simulink model "simple_logic_calculator"  (R2017b)
settings: Solver=FixedStepDiscrete  StartTime=0.0  StopTime=10.0  RelTol=1e-3
settings Model: Creator=ebrah  LastModifiedBy=ebrah
settings OptimizationCC: DefaultParameterBehavior=Inlined  PassReuseOutputArgsAs=Individual arguments
settings DebuggingCC: ParameterTunabilityLossMsg=error
settings SFSimCC: MATLABDynamicMemAlloc=off
settings RTWCC: SystemTargetFile=ert.tlc  GenCodeOnly=on  TemplateMakefile=ert_default_tmf  GenerateReport=on  IncludeHyperlinkInReport=on  LaunchReport=on  GenerateTraceInfo=on  GenerateTraceReport=on  GenerateTraceReportSl=on  GenerateTraceReportSf=on  GenerateTraceReportEml=on  GenerateWebview=on
settings CodeAppCC: ForceParamTrailComments=on  IgnoreCustomStorageClasses=off  OperatorAnnotations=on  SimulinkDataObjDesc=on  SFDataObjDesc=on  InsertBlockDesc=on
settings ERTTargetCC: TargetLangStandard=C99 (ISO)  GenerateSampleERTMain=on  InlinedParameterPlacement=NonHierarchical  ERTCustomFileTemplate=example_file_process.tlc

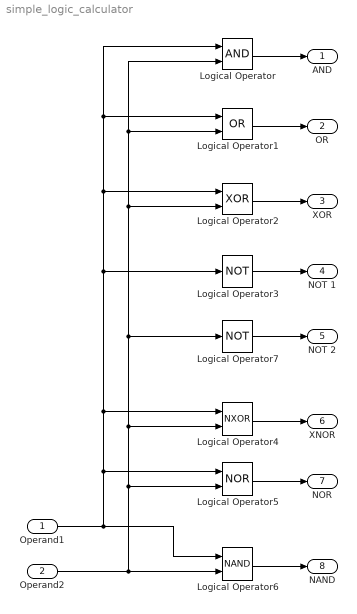
== system simple_logic_calculator ==
  Operand1 : Inport
  Operand2 : Inport  Port=2
  Logical Operator : Logic  AllPortsSameDT=off  OutDataTypeStr=boolean
  Logical Operator1 : Logic  Operator=OR  AllPortsSameDT=off  OutDataTypeStr=boolean
  Logical Operator2 : Logic  Operator=XOR  AllPortsSameDT=off  OutDataTypeStr=boolean
  Logical Operator3 : Logic  Operator=NOT  AllPortsSameDT=off  OutDataTypeStr=boolean
  Logical Operator4 : Logic  Operator=NXOR  AllPortsSameDT=off  OutDataTypeStr=boolean
  Logical Operator5 : Logic  Operator=NOR  AllPortsSameDT=off  OutDataTypeStr=boolean
  Logical Operator6 : Logic  Operator=NAND  AllPortsSameDT=off  OutDataTypeStr=boolean
  Logical Operator7 : Logic  Operator=NOT  AllPortsSameDT=off  OutDataTypeStr=boolean
  AND : Outport
  OR : Outport  Port=2
  XOR : Outport  Port=3
  NOT 1 : Outport  Port=4
  NOT 2 : Outport  Port=5
  XNOR : Outport  Port=6
  NOR : Outport  Port=7
  NAND : Outport  Port=8
  wires:
  Operand1/1 -> Logical Operator3/1, Logical Operator2/1, Logical Operator1/1, Logical Operator/1, Logical Operator4/1, Logical Operator5/1, Logical Operator6/1
  Operand2/1 -> Logical Operator7/1, Logical Operator2/2, Logical Operator1/2, Logical Operator/2, Logical Operator4/2, Logical Operator5/2, Logical Operator6/2
  Logical Operator/1 -> AND/1
  Logical Operator1/1 -> OR/1
  Logical Operator2/1 -> XOR/1
  Logical Operator3/1 -> NOT 1/1
  Logical Operator7/1 -> NOT 2/1
  Logical Operator4/1 -> XNOR/1
  Logical Operator5/1 -> NOR/1
  Logical Operator6/1 -> NAND/1
